simulink model "Model1"  (R2018b)
settings: Solver=VariableStepAuto  StartTime=0.0  StopTime=10.0  RelTol=1e-3
libraries: dspfdesign x2
settings Model: Creator=Fabi Kadir  LastModifiedBy=Fabi Kadir

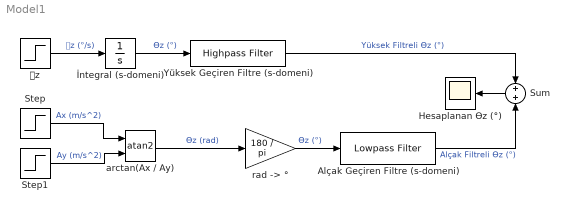
== system Model1 ==
  Alçak Geçiren Filtre (s-domeni) : dspfdesign/Lowpass Filter  FilterType=FIR  DesignForMinimumOrder=on  FilterOrder=50  PassbandFrequency=8e3  StopbandFrequency=12e3  PassbandRipple=0.1  StopbandAttenuation=80  InheritSampleRate=off  SampleRate=44100  SimulateUsing=Interpreted execution  roundingMode=Floor  coeffsDataTypeStr=fixdt(1,16)
  Hesaplanan Өz (°) : Scope
  Step : Step  SampleTime=0
  Step1 : Step  SampleTime=0
  Sum : Sum  Inputs=+|+
  Yüksek Geçiren Filtre (s-domeni) : dspfdesign/Highpass Filter  FilterType=FIR  DesignForMinimumOrder=on  FilterOrder=50  StopbandFrequency=8e3  PassbandFrequency=12e3  StopbandAttenuation=80  PassbandRipple=0.1  InheritSampleRate=off  SampleRate=44100  SimulateUsing=Interpreted execution  roundingMode=Floor  coeffsDataTypeStr=fixdt(1,16)
      settings: SourceProductName=DSP System Toolbox
  arctan(Ax / Ay) : Trigonometry  Operator=atan2
  "rad -> °" : Gain  Gain=180 / pi
  İntegral (s-domeni) : Integrator
  Ꞷz : Step  SampleTime=0
  wires:
  İntegral (s-domeni)/1 -> Yüksek Geçiren Filtre (s-domeni)/1  "Өz (°)"
  Ꞷz/1 -> İntegral (s-domeni)/1  "Ꞷz (°/s)"
  Step/1 -> arctan(Ax / Ay)/1  "Ax (m/s^2)"
  Step1/1 -> arctan(Ax / Ay)/2  "Ay (m/s^2)"
  arctan(Ax / Ay)/1 -> "rad -> °"/1  "Өz (rad)"
  "rad -> °"/1 -> Alçak Geçiren Filtre (s-domeni)/1  "Өz (°)"
  Alçak Geçiren Filtre (s-domeni)/1 -> Sum/2  "Alçak Filtreli Өz (°)"
  Yüksek Geçiren Filtre (s-domeni)/1 -> Sum/1  "Yüksek Filtreli Өz (°)"
  Sum/1 -> Hesaplanan Өz (°)/1
